simulink model "budynek_model"  (R2020b)
settings: Solver=ode4  StartTime=0.0  StopTime=70000  FixedStep=0.1  RelTol=1e-3
model workspace (MAT data in the model file):
  sample_time = 0.1
values from neighbouring files (symbols this model uses):
  cb = 1000    [budynek_zmienne.m]
  ch = 2700    [budynek_zmienne.m]
  cw = 4200    [budynek_zmienne.m]
  dzeta = 1000    [budynek_zmienne.m]
  kext = 15000    [budynek_zmienne.m]
  kh = 12000    [budynek_zmienne.m]
  mb = 20000    [budynek_zmienne.m]
  mh = 3000    [budynek_zmienne.m]
undefined symbols (not defined in the file or in its folder): DiscIntNeverNeededParam
libraries: pid_lib x1
settings Model: Creator=MateuszTg55  LastModifiedBy=mateu
settings OptimizationCC: DefaultParameterBehavior=Inlined  EnhancedBackFolding=on  PassReuseOutputArgsAs=Individual arguments  ZeroExternalMemoryAtStartup=off  ZeroInternalMemoryAtStartup=off  OptimizeBlockOrder=speed  DifferentSizesBufferReuse=on  OptimizationCustomize=off  EfficientTunableParamExpr=on
settings DebuggingCC: ParameterTunabilityLossMsg=error
settings SFSimCC: MATLABDynamicMemAlloc=off
settings RTWCC: Description=Create Visual C/C++ Solution File for Embedded Coder  SystemTargetFile=ert.tlc  GenCodeOnly=on  TemplateMakefile=RTW.MSVCBuild  TargetLang=C++
settings CodeAppCC: ForceParamTrailComments=on  IgnoreCustomStorageClasses=off  OperatorAnnotations=on  SimulinkDataObjDesc=on  SFDataObjDesc=on  InsertBlockDesc=on
settings ERTTargetCC: TargetLangStandard=C++03 (ISO)  GenerateSampleERTMain=on  CodeInterfacePackaging=C++ class  InlinedParameterPlacement=NonHierarchical  RootIOFormat=Structure reference  ERTCustomFileTemplate=example_file_process.tlc

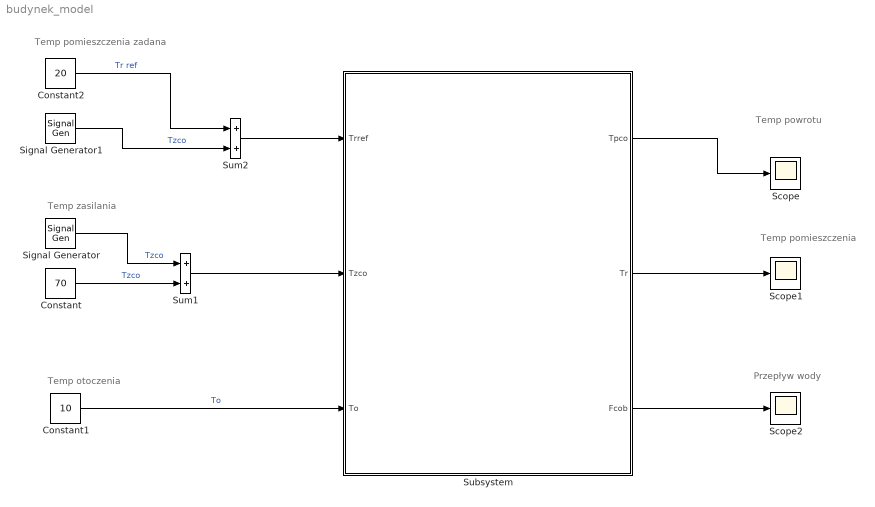
== system budynek_model ==
  note: Przepływ wody
  note: Temp otoczenia
  note: Temp pomieszczenia zadana
  note: Temp powrotu
  note: Temp zasilania
  note: Temp pomieszczenia
  Constant : Constant  Value=70
  Constant1 : Constant  Value=10
  Constant2 : Constant  Value=20
  Scope : Scope
  Scope1 : Scope
  Scope2 : Scope
  Signal Generator : SignalGenerator  WaveForm=square  Amplitude=10  Frequency=0.001
  Signal Generator1 : SignalGenerator  WaveForm=square  Amplitude=10  Frequency=0.00002
  Subsystem : Subsystem  TreatAsAtomicUnit=on  SystemSampleTime=sample_time
  Sum1 : Sum
  Sum2 : Sum
  wires:
  Constant2/1 -> Sum2/1  "Tr ref"
  Constant/1 -> Sum1/2  "Tzco"
  Sum2/1 -> Subsystem/1(Trref)
  Sum1/1 -> Subsystem/2(Tzco)
  Constant1/1 -> Subsystem/3(To)  "To"
  Subsystem/1(Tpco) -> Scope/1
  Subsystem/2(Tr) -> Scope1/1
  Signal Generator1/1 -> Sum2/2  "Tzco"
  Signal Generator/1 -> Sum1/1  "Tzco"
  Subsystem/3(Fcob) -> Scope2/1

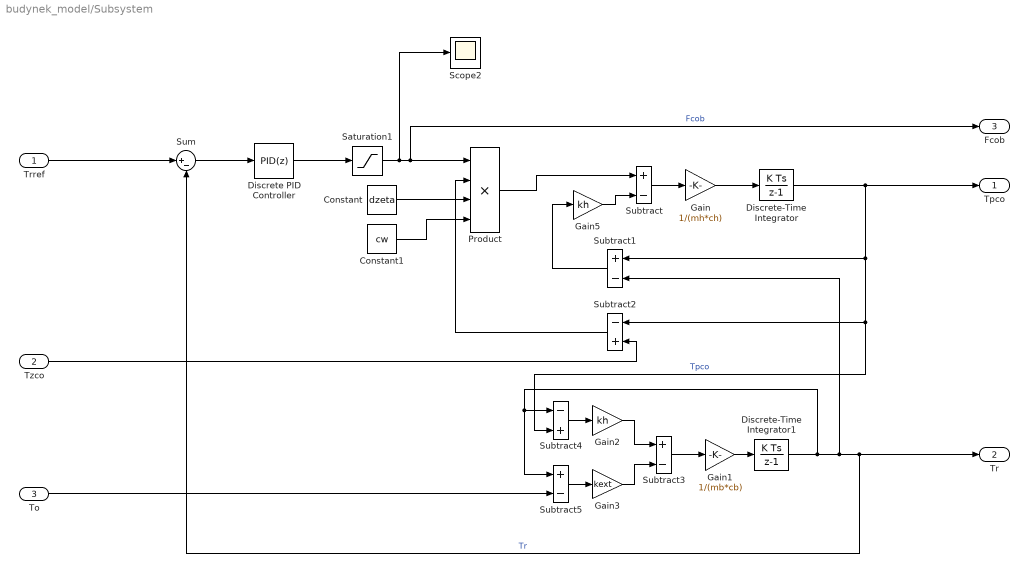
== system budynek_model/Subsystem ==
  Trref : Inport
  Tzco : Inport  Port=2
  To : Inport  Port=3
  Constant : Constant  Value=dzeta
  Constant1 : Constant  Value=cw
  Discrete PID Controller : pid_lib/PID Controller  Controller=PID  Form=Parallel  TimeDomain=Discrete-time  UseExternalTs=off  SampleTime=sample_time  IntegratorMethod=Forward Euler  FilterMethod=Forward Euler  ControllerParametersSource=internal  P=0.000316420719124277  I=1.42804500861683e-07  D=-0.00168554182386  UseFilter=on  N=0.171582409720465  TunerSelectOption=Transfer Function Based (PID Tuner App)  InitialConditionSource=internal  InitialConditionForIntegrator=0  InitialConditionForFilter=0  DifferentiatorICPrevScaledInput=0  ExternalReset=none  TrackingMode=off  Kt=1  LimitOutput=off  SatLimitsSource=internal  UpperSaturationLimit=inf  LowerSaturationLimit=-inf  LinearizeAsGain=off  AntiWindupMode=none  Kb=1  POutMin=[]  POutMax=[]  IOutMin=[]  IOutMax=[]  DOutMin=[]  DOutMax=[]  NOutMin=[]  NOutMax=[]  SumOutMin=[]  SumOutMax=[]  SaturationOutMin=[]  SaturationOutMax=[]  PParamMin=[]  PParamMax=[]  IParamMin=[]  IParamMax=[]  DParamMin=[]  DParamMax=[]  NParamMin=[]  NParamMax=[]  KbParamMin=[]  KbParamMax=[]  KtParamMin=[]  KtParamMax=[]  KbOutMin=[]  KbOutMax=[]  KtOutMin=[]  KtOutMax=[]  IntegratorOutMin=[]  IntegratorOutMax=[]  FilterOutMin=[]  FilterOutMax=[]  SumI1OutMin=[]  SumI1OutMax=[]  SumI2OutMin=[]  SumI2OutMax=[]  SumI3OutMin=[]  SumI3OutMax=[]  SumI4OutMin=[]  SumI4OutMax=[]  SumDOutMin=[]  SumDOutMax=[]  DifferentiatorOutMin=[]  DifferentiatorOutMax=[]  FilterDiffOutCoefMin=[]  FilterDiffOutCoefMax=[]  ReciprocalOutMin=[]  ReciprocalOutMax=[]  SumDenOutMin=[]  SumDenOutMax=[]  SumNumOutMin=[]  SumNumOutMax=[]  DivideOutMin=[]  DivideOutMax=[]  UdiffTsProdOutMin=[]  UdiffTsProdOutMax=[]  NTsProdOutMin=[]  NTsProdOutMax=[]  UintegralTsProdOutMin=[]  UintegralTsProdOutMax=[]  UngainTsProdOutMin=[]  UngainTsProdOutMax=[]  IntegratorContinuousStateAttributes=''  IntegratorStateMustResolveToSignalObject=off  IntegratorRTWStateStorageClass=Auto  FilterContinuousStateAttributes=''  FilterStateMustResolveToSignalObject=off  FilterRTWStateStorageClass=Auto  ParallelPVariant=InternalParameters  IdealPVariant=Disabled  IVariant=InternalParameters  DVariant=InternalParameters  IntegratorVariant=Discrete  SatVariant=Disabled  AWVariant=Passthrough  PCopyVariant=Disabled  TRVariant=Disabled  FdbkBlocksVariant=Forward  IdealPFdbkVariant=Disabled  SatFdbkVariant=Disabled  DerivativeFilterVariant=ForwardEulerFilter  NVariant=InternalParameters  NCopyVariant=Disabled  FilterICVariant=InternalICsFilter  IntegratorICVariant=InternalICs  ExternalResetVariant=Disabled  TRSumVariant=Passthrough  SumFdbkVariant=Disabled  SumVariant=Sum_PID  TsampFilterVariant=InternalTs  TsampNgainVariant=Passthrough  TsampIntegralVariant=Passthrough  ExternalSaturationOutDataTypeStr=Inherit: Same as second input
  Discrete-Time Integrator : DiscreteIntegrator  InitialCondition=22  SampleTime=sample_time  ICPrevOutput=DiscIntNeverNeededParam  ICPrevScaledInput=DiscIntNeverNeededParam
  Discrete-Time Integrator1 : DiscreteIntegrator  InitialCondition=15  SampleTime=sample_time  ICPrevOutput=DiscIntNeverNeededParam  ICPrevScaledInput=DiscIntNeverNeededParam
  Gain : Gain  Gain=1/(mh*ch)
  Gain1 : Gain  Gain=1/(mb*cb)
  Gain2 : Gain  Gain=kh
  Gain3 : Gain  Gain=kext
  Gain5 : Gain  Gain=kh
  Product : Product  Inputs=4
  Saturation1 : Saturate  UpperLimit=30/3600  LowerLimit=0
  Scope2 : Scope
  Subtract{,1,3,5} (4 alike) : Sum  Inputs=+-
  Subtract2 : Sum  Inputs=-+
  Subtract4 : Sum  Inputs=-+
  Sum : Sum  Inputs=|+-
  Tpco : Outport
  Tr : Outport  Port=2
  Fcob : Outport  Port=3
  wires:
  Gain/1 -> Discrete-Time Integrator/1
  Gain3/1 -> Subtract3/2
  Discrete-Time Integrator1/1 -> Tr/1, Sum/2, Subtract1/2, Subtract5/1, Subtract4/1  "Tr"
  Discrete-Time Integrator/1 -> Subtract4/2, Subtract2/1, Subtract1/1, Tpco/1  "Tpco"
  Saturation1/1 -> Product/1, Fcob/1, Scope2/1  "Fcob"
  Subtract/1 -> Gain/1
  Discrete PID Controller/1 -> Saturation1/1
  Gain1/1 -> Discrete-Time Integrator1/1
  Sum/1 -> Discrete PID Controller/1
  Subtract4/1 -> Gain2/1
  Subtract3/1 -> Gain1/1
  Gain2/1 -> Subtract3/1
  Trref/1 -> Sum/1
  Subtract5/1 -> Gain3/1
  Subtract1/1 -> Gain5/1
  Gain5/1 -> Subtract/2
  Tzco/1 -> Subtract2/2
  Subtract2/1 -> Product/2
  To/1 -> Subtract5/2
  Constant/1 -> Product/3
  Constant1/1 -> Product/4
  Product/1 -> Subtract/1
